simulink model "Helicopter_NL_Data"  (R2018a)
settings: Solver=VariableStepAuto  StartTime=0.0  StopTime=inf  RelTol=1e-3
undefined symbols (not defined in the file or in its folder): daq
libraries: daqlib x2, realtime_pacer_lib x1
settings Model: Creator=pacoa  LastModifiedBy=pacoa

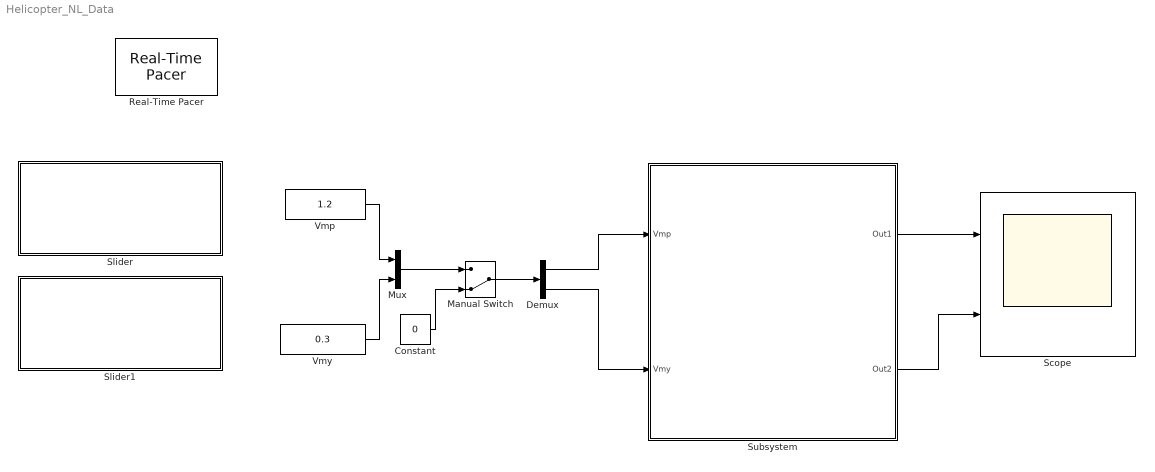
== system Helicopter_NL_Data ==
  Constant : Constant  Value=0
  Demux : Demux  Outputs=2
  Manual Switch : ManualSwitch  CurrentSetting=0
  Mux : Mux  Inputs=2
  Real-Time Pacer : realtime_pacer_lib/Real-Time Pacer  simTimePerRealTime=10
  Scope : Scope  NumInputPorts=2
  Slider : Subsystem  DialogController=hmiCreateDDGDialog  IsWebBlock=on  mask(MWDashboardBlock){webBlockId=304629f1-18d4-497e-8737-874cc7ed481c, webBlockType=slider, ShowInLibBrowser=on, ShowInitialText=on, HMISrcModelName=Helicopter_NL_Data}
      mask prompts: webBlockId "WebBlock Id"; webBlockType "WebBlock Type"; HMISrcModelName "Source Model"
      mask help: SimulinkHMI:dialogs:SliderDialogDesc
      mask Help: helpview([docroot '/mapfiles/simulink.map'], 'hmi_slider')
      mask Display:
      | if strcmp(get_param(bdroot(gcb),'BlockDiagramType'), 'library')
      |     image([(matlabroot) '/toolbox/simulink/hmi/icons/Slider.png']);
      | end
  Slider1 : Subsystem  DialogController=hmiCreateDDGDialog  IsWebBlock=on  mask(MWDashboardBlock){webBlockId=ef8de569-e3ff-48d1-b0e4-6efc81bd23b0, webBlockType=slider, ShowInLibBrowser=on, ShowInitialText=on, HMISrcModelName=Helicopter_NL_Data}
      mask prompts: webBlockId "WebBlock Id"; webBlockType "WebBlock Type"; HMISrcModelName "Source Model"
      mask help: SimulinkHMI:dialogs:SliderDialogDesc
      mask Help: helpview([docroot '/mapfiles/simulink.map'], 'hmi_slider')
      mask Display:
      | if strcmp(get_param(bdroot(gcb),'BlockDiagramType'), 'library')
      |     image([(matlabroot) '/toolbox/simulink/hmi/icons/Slider.png']);
      | end
  Subsystem : Subsystem
  Vmp : Constant  Value=1.2
  Vmy : Constant  Value=0.3
  wires:
  Subsystem/1(Out1) -> Scope/1
  Vmy/1 -> Mux/2
  Vmp/1 -> Mux/1
  Mux/1 -> Manual Switch/1
  Constant/1 -> Manual Switch/2
  Manual Switch/1 -> Demux/1
  Demux/1 -> Subsystem/1(Vmp)
  Demux/2 -> Subsystem/2(Vmy)
  Subsystem/2(Out2) -> Scope/2

== system Helicopter_NL_Data/Slider ==

== system Helicopter_NL_Data/Slider1 ==

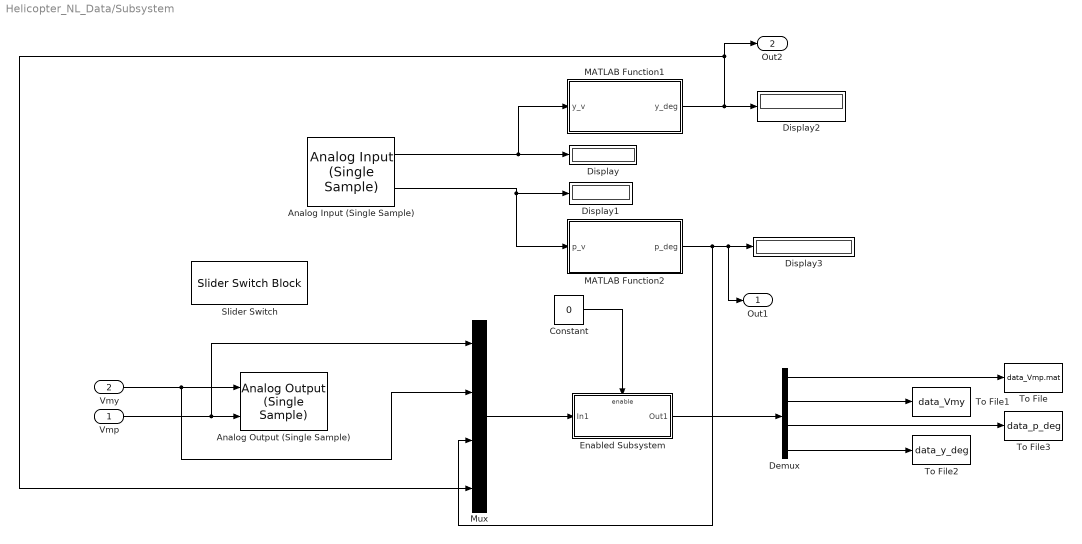
== system Helicopter_NL_Data/Subsystem ==
  Vmp : Inport
  Vmy : Inport  Port=2
  Analog Input (Single Sample) : daqlib/Analog Input (Single Sample)  DeviceMenu=ni Dev4 (USB-6001)  Device=ni Dev4 (USB-6001)  ObjConstructor=daq.createSession('ni')  BlockSampleTime=-1  NChannelsSelected=2  Channels=1$ai0$$Dev4$1$1$2$1$#1$ai1$$Dev4$1$1$2$1$#0$ai2$$Dev4$1$1$2$1$#0$ai3$$Dev4$1$1$2$1$#0$ai4$$Dev4$1$1$1$1$#0$ai5$$Dev4$1$1$1$1$#0$ai6$$Dev4$1$1$1$1$#0$ai7$$Dev4$1$1$1$1$#  NPorts=1 per channel  OutputTimestamp=off
      settings: SourceProductName=Data Acquisition Toolbox  SourceProductBaseCode=DA
  Analog Output (Single Sample) : daqlib/Analog Output (Single Sample)  DeviceMenu=ni Dev4 (USB-6001)  Device=ni Dev4 (USB-6001)  ObjConstructor=daq.createSession('ni')  NChannelsSelected=2  Channels=1$ao0$$Dev4$1$1$N/A$#1$ao1$$Dev4$1$1$N/A$#  NPorts=1 per channel  BlockSampleTime=-1
      settings: SourceProductName=Data Acquisition Toolbox  SourceProductBaseCode=DA
  Constant : Constant  Value=0
  Demux : Demux
  Display{,1..3} (4 alike) : Display
  Enabled Subsystem : Subsystem  TreatAsAtomicUnit=on
  MATLAB Function1 : MATLAB Function  TreatAsAtomicUnit=on
  MATLAB Function2 : MATLAB Function  TreatAsAtomicUnit=on
  Mux : Mux
  Slider Switch : SliderSwitchBlock  WebBlockId=68
      settings: Values={{'Off', 'On'}, [0 1]}
  To File : ToFile  Filename=data_Vmp.mat  MatrixName=Vmp_meas  SaveFormat=Timeseries
  To File1 : ToFile  Filename=data_Vmy  MatrixName=Vmy_meas  SaveFormat=Timeseries
  To File2 : ToFile  Filename=data_y_deg  MatrixName=y_deg_meas  SaveFormat=Timeseries
  To File3 : ToFile  Filename=data_p_deg  MatrixName=p_deg  SaveFormat=Timeseries
  Out1 : Outport
  Out2 : Outport  Port=2
  wires:
  MATLAB Function1/1(y_deg) -> Display2/1, Mux/4, Out2/1
  Analog Input (Single Sample)/1 -> Display/1, MATLAB Function1/1(y_v)
  MATLAB Function2/1(p_deg) -> Mux/3, Display3/1, Out1/1
  Analog Input (Single Sample)/2 -> Display1/1, MATLAB Function2/1(p_v)
  Constant/1 -> Enabled Subsystem/Enable
  Vmy/1 -> Mux/2, Analog Output (Single Sample)/1
  Vmp/1 -> Analog Output (Single Sample)/2, Mux/1
  Mux/1 -> Enabled Subsystem/1(In1)
  Enabled Subsystem/1(Out1) -> Demux/1
  Demux/1 -> To File/1
  Demux/2 -> To File1/1
  Demux/3 -> To File3/1
  Demux/4 -> To File2/1

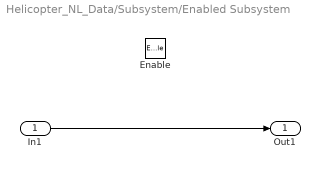
== system Helicopter_NL_Data/Subsystem/Enabled Subsystem ==
  In1 : Inport
  Enable : EnablePort
  Out1 : Outport
  wires:
  In1/1 -> Out1/1

== matlab function Helicopter_NL_Data/Subsystem/MATLAB Function1 ==
  data: y_v input size=[1]; y_deg output size=[1]
function y_deg = y_V_to_deg(y_v)
error = 0.145;
y_v = y_v -error;
V_max = 5;
V_min = 0;
deg_max = 180;
deg_min = 0;
m =(deg_max - deg_min)/(V_max - V_min)
y_deg = m*(y_v -V_min) + deg_min;

== matlab function Helicopter_NL_Data/Subsystem/MATLAB Function2 ==
  data: p_v input size=[1]; p_deg output size=[1]
function p_deg = p_V_to_deg(p_v)
error = 0.12;
p_v = p_v - error;
V_max = 5;
V_min = 0;
deg_max = 45;
deg_min = -45;
m =(deg_max - deg_min)/(V_max - V_min)
p_deg = m*(p_v -V_min) + deg_min;
